simulink model "1- ISI_ideal_system"  (R2018a)
settings: Solver=VariableStepDiscrete  StartTime=0.0  StopTime=L  RelTol=1e-3  EnableMultiTasking=on
values from neighbouring files (symbols this model uses):
  N = 20    [0- ISI_init.m]
  T = 1e-3    (= 0.001)    [0- ISI_init.m]
libraries: simulink x3, commrandsrc2 x1
settings Model: Creator=calin  LastModifiedBy=Ahmed Saleh
settings DataIOCC: LimitDataPoints=on  SaveFormat=Array  SignalLoggingSaveFormat=ModelDataLogs
settings OptimizationCC: InitFltsAndDblsToZero=on  LifeSpan=inf
settings DebuggingCC: SaveWithParameterizedLinksMsg=none  UnderspecifiedInitializationDetection=Classic  MergeDetectMultiDrivingBlocksExec=none  SignalResolutionControl=TryResolveAllWithWarning  SolverPrmCheckMsg=warning  MultiTaskDSMMsg=warning  MultiTaskCondExecSysMsg=none  FcnCallInpInsideContextMsg=warning  StateNameClashWarn=warning  SFUnexpectedBacktrackingDiag=warning  SFNoUnconditionalDefaultTransitionDiag=warning  SFExecutionAtInitializationDiag=none
settings HardwareCC: ProdBitPerPointer=32  ProdBitPerSizeT=32  ProdBitPerPtrDiffT=32  ProdLargestAtomicFloat=None  ProdIntDivRoundTo=Undefined  ProdEndianess=Unspecified  ProdWordSize=32  ProdHWDeviceType=32-bit Generic
settings ModelReferenceCC: PropagateSignalLabelsOutOfModel=off
settings CodeAppCC: StateflowObjectComments=on
settings GRTTargetCC: TargetFcnLib=ansi_tfl_tmw.mat  TargetLangStandard=C89/C90 (ANSI)  CombineOutputUpdateFcns=off  GRTInterface=on
settings ConfigComp: CovMetricSettings=dw  CovHtmlReporting=on  CovSaveCumulativeToWorkspaceVar=on  CovSaveSingleToWorkspaceVar=on  CovExternalEMLEnable=off

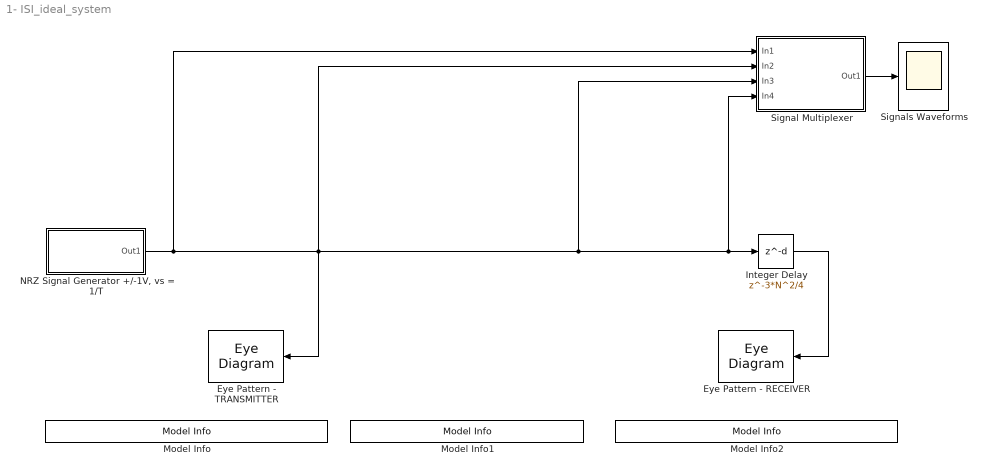
== system 1- ISI_ideal_system ==
  Eye Pattern - RECEIVER : EyeDiagram  Tag=EyeDiagram
  Eye Pattern - TRANSMITTER : EyeDiagram  Tag=EyeDiagram
  Integer Delay : Delay  DelayLength=3*N^2/4  InputProcessing=Inherited
  Model Info : simulink/Model-Wide Utilities/Model Info  Frame=on  DisplayStringWithTags=TRANSMITTER  HorizontalTextAlignment=Center  LeftAlignmentValue=0.5
  Model Info1 : simulink/Model-Wide Utilities/Model Info  Frame=on  DisplayStringWithTags=CHANNEL MODEL  HorizontalTextAlignment=Center  LeftAlignmentValue=0.5
  Model Info2 : simulink/Model-Wide Utilities/Model Info  Frame=on  DisplayStringWithTags=RECEIVER  HorizontalTextAlignment=Center  LeftAlignmentValue=0.5
  "NRZ Signal Generator +/-1V, vs = 1/T" : Subsystem
  Signal Multiplexer : Subsystem
  Signals Waveforms : Scope
  wires:
  "NRZ Signal Generator +/-1V, vs = 1/T"/1(Out1) -> Integer Delay/1, Signal Multiplexer/4(In4), Signal Multiplexer/3(In3), Eye Pattern - TRANSMITTER/1, Signal Multiplexer/2(In2), Signal Multiplexer/1(In1)
  Integer Delay/1 -> Eye Pattern - RECEIVER/1
  Signal Multiplexer/1(Out1) -> Signals Waveforms/1

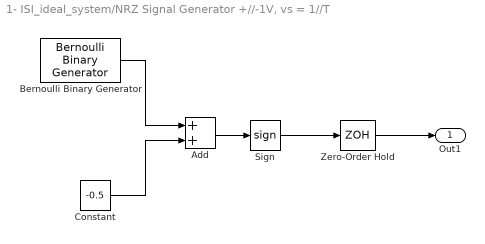
== system 1- ISI_ideal_system/NRZ Signal Generator +//-1V, vs = 1//T ==
  Add : Sum
  Bernoulli Binary Generator : commrandsrc2/Bernoulli Binary Generator  P=0.5  seed=61  Ts=T  frameBased=off  sampPerFrame=1  orient=off  outDataType=double
  Constant : Constant  Value=-0.5
  Sign : Signum  ZeroCross=off
  Zero-Order Hold : ZeroOrderHold  SampleTime=-1
  Out1 : Outport
  wires:
  Zero-Order Hold/1 -> Out1/1
  Sign/1 -> Zero-Order Hold/1
  Bernoulli Binary Generator/1 -> Add/1
  Add/1 -> Sign/1
  Constant/1 -> Add/2

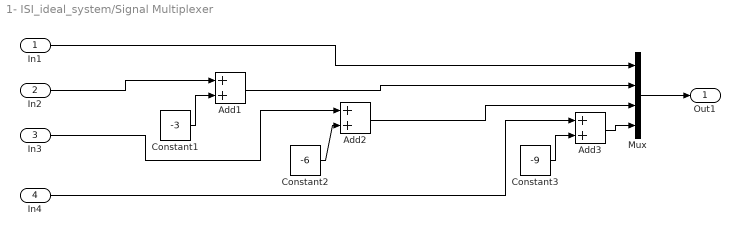
== system 1- ISI_ideal_system/Signal Multiplexer ==
  In1 : Inport
  In2 : Inport  Port=2
  In3 : Inport  Port=3
  In4 : Inport  Port=4
  Add1 : Sum
  Add2 : Sum
  Add3 : Sum
  Constant1 : Constant  Value=-3
  Constant2 : Constant  Value=-6
  Constant3 : Constant  Value=-9
  Mux : Mux
  Out1 : Outport
  wires:
  Mux/1 -> Out1/1
  Constant1/1 -> Add1/2
  Add1/1 -> Mux/2
  Constant2/1 -> Add2/2
  Add2/1 -> Mux/3
  Constant3/1 -> Add3/2
  Add3/1 -> Mux/4
  In1/1 -> Mux/1
  In2/1 -> Add1/1
  In3/1 -> Add2/1
  In4/1 -> Add3/1
